simulink model "L0504"  (Simulink 9.1)
settings: Solver=ode45  StartTime=0.0  StopTime=80  MaxStep=0.1  RelTol=1e-3
libraries: simulink x2
settings Model: Creator=Asus  LastModifiedBy=Asus
settings DataIOCC: SaveFormat=Dataset
settings OptimizationCC: LifeSpan=auto
settings DebuggingCC: UnderspecifiedInitializationDetection=Simplified  MergeDetectMultiDrivingBlocksExec=error  SFUnexpectedBacktrackingDiag=error  SFNoUnconditionalDefaultTransitionDiag=error  SFExecutionAtInitializationDiag=warning
settings HardwareCC: ProdBitPerPointer=64  ProdBitPerSizeT=64  ProdBitPerPtrDiffT=64  ProdLargestAtomicFloat=Float  ProdIntDivRoundTo=Zero  ProdEndianess=LittleEndian  ProdWordSize=64  ProdHWDeviceType=Intel->x86-64 (Windows64)
settings ModelReferenceCC: PropagateSignalLabelsOutOfModel=on
settings CodeAppCC: StateflowObjectComments=off
settings GRTTargetCC: TargetLangStandard=C99 (ISO)  CombineOutputUpdateFcns=on  GRTInterface=off
settings ConfigComp: CovMetricSettings=dwe  CovHtmlReporting=off  CovSaveCumulativeToWorkspaceVar=off  CovSaveSingleToWorkspaceVar=off  CovExternalEMLEnable=on

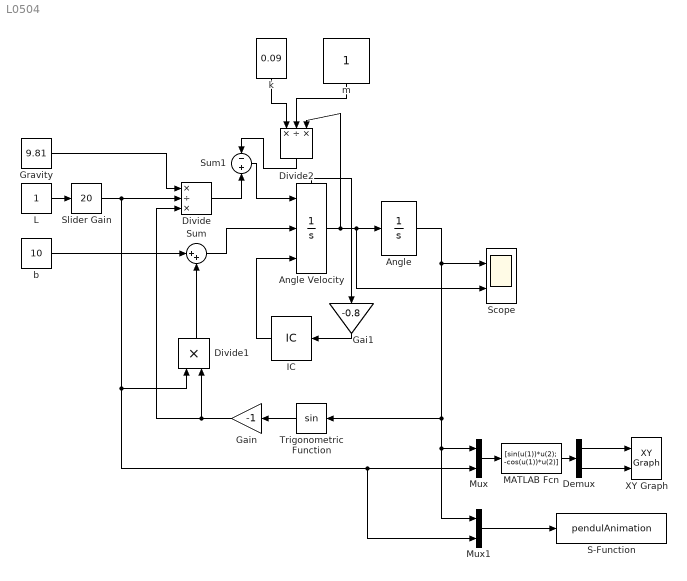
== system L0504 ==
  Angle : Integrator
  Angle Velocity : Integrator  ExternalReset=either  InitialConditionSource=external  InitialCondition=1  ShowStatePort=on
  Demux : Demux  Outputs=2
  Divide : Product  Inputs=*/*
  Divide1 : Product  Inputs=**
  Divide2 : Product  Inputs=*/*
  Gai1 : Gain  Gain=-0.8
  Gain : Gain  Gain=-1
  Gravity : Constant  Value=9.81
  IC : InitialCondition  Value=2
  L : Constant
  MATLAB Fcn : MATLABFcn  MATLABFcn=[sin(u(1))*u(2); -cos(u(1))*u(2)]
  Mux : Mux  Inputs=2
  Mux1 : Mux  Inputs=2
  S-Function : S-Function  FunctionName=pendulAnimation  Parameters=0.1  SFunctionDeploymentMode=off  EnableBusSupport=off
  Scope : Scope  NumInputPorts=2
  Slider Gain : simulink/Math Operations/Slider Gain  gain=20  low=0  high=50
  Sum : Sum  Inputs=|++
  Sum1 : Sum  Inputs=-+
  Trigonometric Function : Trigonometry
  XY Graph : simulink/Sinks/XY Graph  xmin=-35  xmax=35  ymin=-35  ymax=35  st=-1
  b : Constant  Value=10
  k : Constant  Value=0.09
  m : Constant
  wires:
  MATLAB Fcn/1 -> Demux/1
  Divide1/1 -> Sum/2
  Angle/1 -> Scope/1, Trigonometric Function/1, Mux1/1, Mux/1
  Divide/1 -> Sum1/2
  Demux/2 -> XY Graph/2
  Gravity/1 -> Divide/1
  IC/1 -> Angle Velocity/3
  Divide2/1 -> Sum1/1
  Sum/1 -> Angle Velocity/2
  k/1 -> Divide2/1
  Gai1/1 -> IC/1
  Sum1/1 -> Angle Velocity/1
  m/1 -> Divide2/2
  Angle Velocity/State -> Gai1/1
  Slider Gain/1 -> Divide/2, Mux1/2, Mux/2, Divide1/1
  b/1 -> Sum/1
  Demux/1 -> XY Graph/1
  Mux/1 -> MATLAB Fcn/1
  Angle Velocity/1 -> Angle/1, Scope/2, Divide2/3
  L/1 -> Slider Gain/1
  Gain/1 -> Divide/3, Divide1/2
  Trigonometric Function/1 -> Gain/1
  Mux1/1 -> S-Function/1
